simulink model "RollAxisAutopilotHarness"  (R2026a)
settings: Solver=FixedStepDiscrete  StartTime=0  StopTime=30  FixedStep=0.025
model workspace (MATLAB code in the model file):
  | cmdLim = Simulink.Parameter;
  | cmdLim.Value = 15;
  | cmdLim.Description = 'Limit for controlling the maximum surface command angle.';
  | cmdLim.Min = 0;
  | cmdLim.Max = 90;
  | cmdLim.DocUnits = 'deg';
  | 
  | dispGain = Simulink.Parameter;
  | dispGain.Value = 0.75;
  | dispGain.Description = 'Gain applied to the displacement error.';
  | dispGain.Min = 0;
  | dispGain.Max = [];
  | dispGain.DocUnits = 'deg/sec/deg';
  | 
  | dispLim = Simulink.Parameter;
  | dispLim.Value = 30;
  | dispLim.Description = 'Limit for controlling the maximum commanded angle.';
  | dispLim.Min = 0;
  | dispLim.Max = 180;
  | dispLim.DocUnits = 'deg';
  | 
  | intGain = Simulink.Parameter;
  | intGain.Value = 0.5;
  | intGain.Description = 'Gain applied to the integral error.';
  | intGain.Min = 0;
  | intGain.Max = [];
  | intGain.DocUnits = 'deg/sec/deg/sec';
  | 
  | intLim = Simulink.Parameter;
  | intLim.Value = 5;
  | intLim.Description = 'Limit for controlling the maximum commanded angle.';
  | intLim.Min = 0;
  | intLim.Max = 90;
  | intLim.DocUnits = 'deg';
  | 
  | rateGain = Simulink.Parameter;
  | rateGain.Value = 2;
  | rateGain.Description = 'Gain applied to the rate error.';
  | rateGain.Min = 0;
  | rateGain.Max = [];
  | rateGain.DocUnits = 'deg/deg/sec';
  | 
  | rateLim = Simulink.Parameter;
  | rateLim.Value = 6;
  | rateLim.Description = 'Limit for controlling the maximum commanded angle.';
  | rateLim.Min = 0;
  | rateLim.Max = 180;
  | rateLim.DocUnits = 'deg/sec';
  | 
  | hdgGain = Simulink.Parameter;
  | hdgGain.Value = 0.015;
libraries: SignalEditorBlockLib x1
settings Model: RequirementInfo={} %GIDa_fe9045fd_0412_4b6e_8206_617cc20e6fde  FPTRunName=Active  SldvGeneratedHarnessModel=TestUnitModel=rtwdemo_roll|  ModifiedByFormat=The MathWorks, Inc.  Creator=The MathWorks, Inc.  LastModifiedBy=The MathWorks, Inc.
settings DataIOCC: ExternalInput=xin  SaveFormat=StructureWithTime  OutputSaveName=harness_yout
settings OptimizationCC: UseDivisionForNetSlopeComputation=on  UseFloatMulNetSlope=on  InlineInvariantSignals=on  ExpressionFolding=off  StateBitsets=on  DataBitsets=on  EfficientFloat2IntCast=on  EfficientMapNaN2IntZero=off  MaxStackSize=inf
settings DebuggingCC: SignalRangeChecking=error  ReadBeforeWriteMsg=EnableAllAsError  WriteAfterWriteMsg=EnableAllAsError  WriteAfterReadMsg=EnableAllAsError  AlgebraicLoopMsg=error  ArtificialAlgebraicLoopMsg=error  SaveWithDisabledLinksMsg=error  SaveWithParameterizedLinksMsg=error  CheckExecutionContextPreStartOutputMsg=on  BlockPriorityViolationMsg=error  MaxConsecutiveZCsMsg=warning  SolverPrmCheckMsg=error  InheritedTsInSrcMsg=none  SingleTaskRateTransMsg=error  TasksWithSamePriorityMsg=error  SigSpecEnsureSampleTimeMsg=error  IntegerOverflowMsg=none  ParameterUnderflowMsg=error  ParameterPrecisionLossMsg=none  UnderSpecifiedDataTypeMsg=error  UnnecessaryDatatypeConvMsg=warning  VectorMatrixConversionMsg=error  SignalLabelMismatchMsg=error  UnconnectedInputMsg=error  UnconnectedOutputMsg=error  UnconnectedLineMsg=error  SFcnCompatibilityMsg=error  UniqueDataStoreMsg=error  BusObjectLabelMismatch=error  RootOutportRequireBusObject=error  AssertControl=DisableAll  ModelReferenceIOMismatchMessage=error  UnknownTsInhSupMsg=error  ModelReferenceDataLoggingMessage=error  ModelReferenceSymbolNameMessage=none  StrictBusMsg=ErrorOnBusTreatedAsVector  BusNameAdapt=ErrorWithoutRepair  NonBusSignalsTreatedAsBus=error  IntegerSaturationMsg=none
settings HardwareCC: TargetBitPerPointer=64.0  TargetBitPerSizeT=64.0  TargetBitPerPtrDiffT=64.0  TargetLongLongMode=on  TargetIntDivRoundTo=Zero  TargetEndianess=LittleEndian  TargetWordSize=64.0  TargetHWDeviceType=Custom Processor->MATLAB Host Computer  ProdEqTarget=off
settings RTWCC: SystemTargetFile=ert.tlc  GenerateReport=on  RTWVerbose=off  IncludeHyperlinkInReport=on  LaunchReport=on  Description=Embedded Coder
settings CodeAppCC: MATLABFcnDesc=on  MATLABSourceComments=on  EnableCustomComments=on  ReqsInCode=on
settings ERTTargetCC: DynamicArrayContainerType=coder::array  UtilityFuncGeneration=Shared location  MultiwordLength=2048.0  GenerateSampleERTMain=on  SupportContinuousTime=on
settings ConfigComp: CovSaveName=covdata_rollAP  CovMetricSettings=dcm  CovHTMLOptions=-sRT=1 -aTS=1 -bRG=1 -bTC=0 -hTR=0 -nFC=0 -scm=1 -bcm=1 -xEv=0  CovCumulativeVarName=covCumulativeData_rollAP  CovReportOnPause=off  DVMaxProcessTime=300.0  DVModelCoverageObjectives=MCDC  DVMaxTestCaseSteps=500.0  DVTestSuiteOptimization=Auto  DVAbsoluteTolerance=1.0e-5  DVDefectChecker=off  DVDetectActiveLogic=on  DVMaxViolationSteps=20.0  DVSaveHarnessModel=on  DVModelReferenceHarness=on  DVHarnessSource=Signal Editor  DVSaveReport=on  DVRebuildModelRepresentation=Always  DVActiveTab=0.0

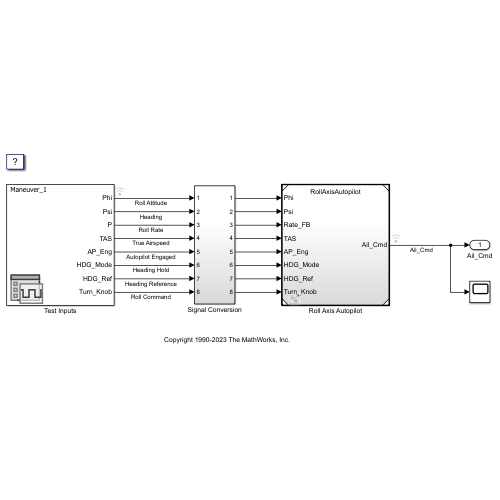
[thumbnail: Simulink's stored preview of the top-level diagram]
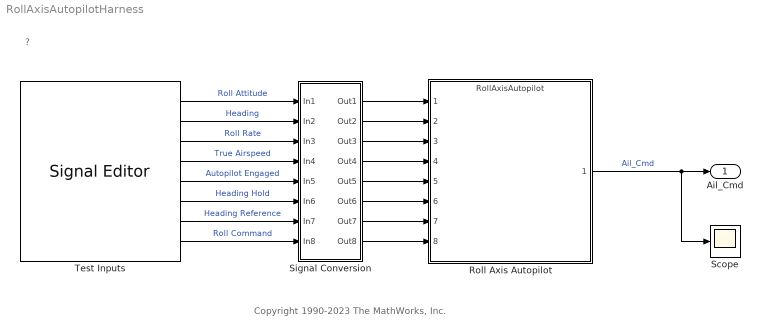
== system RollAxisAutopilotHarness ==
  note: Copyright 1990-2023 The MathWorks, Inc.
  note: ?
  Roll Axis Autopilot : ModelReference  ModelNameDialog=RollAxisAutopilot.slx  SimulationMode=Normal  ModelReferenceVersion=13.1
  Scope : Scope
      settings: DataLoggingSaveFormat=Array
  Signal Conversion : Subsystem
  Test Inputs : SignalEditorBlockLib/Signal Editor  FileName=roll_harness_TestInputs.mat  ActiveScenario=Maneuver_1  ActiveSignal=Turn_Knob  IsBus=off  OutputBusObjectStr=Bus: BusObject  SampleTime=0  ZeroCross=off  OutputAfterFinalValue=Extrapolation  Unit=inherit  PreserveSignalName=off  ApplySigPropsToAllScenarios=on  ApplySigPropsToAllSignals=off  SignalPropertySource=Dialog parameters
  Ail_Cmd : Outport  RequirementInfo={} %GIDa_7d37a828_8c9c_441a_973a_3dcc496ec4f2  OutMin=-15  OutMax=15  OutDataTypeStr=single  PortDimensions=1  SampleTime=1/40  VectorParamsAs1DForOutWhenUnconnected=off
  wires:
  Test Inputs/1 -> Signal Conversion/1(In1)  "Roll Attitude"
  Signal Conversion/1(Out1) -> Roll Axis Autopilot/1
  Test Inputs/2 -> Signal Conversion/2(In2)  "Heading"
  Signal Conversion/2(Out2) -> Roll Axis Autopilot/2
  Test Inputs/3 -> Signal Conversion/3(In3)  "Roll Rate"
  Signal Conversion/3(Out3) -> Roll Axis Autopilot/3
  Test Inputs/4 -> Signal Conversion/4(In4)  "True Airspeed"
  Signal Conversion/4(Out4) -> Roll Axis Autopilot/4
  Test Inputs/5 -> Signal Conversion/5(In5)  "Autopilot Engaged"
  Signal Conversion/5(Out5) -> Roll Axis Autopilot/5
  Test Inputs/6 -> Signal Conversion/6(In6)  "Heading Hold"
  Signal Conversion/6(Out6) -> Roll Axis Autopilot/6
  Test Inputs/7 -> Signal Conversion/7(In7)  "Heading Reference"
  Signal Conversion/7(Out7) -> Roll Axis Autopilot/7
  Test Inputs/8 -> Signal Conversion/8(In8)  "Roll Command"
  Signal Conversion/8(Out8) -> Roll Axis Autopilot/8
  Roll Axis Autopilot/1 -> Scope/1, Ail_Cmd/1  "Ail_Cmd"

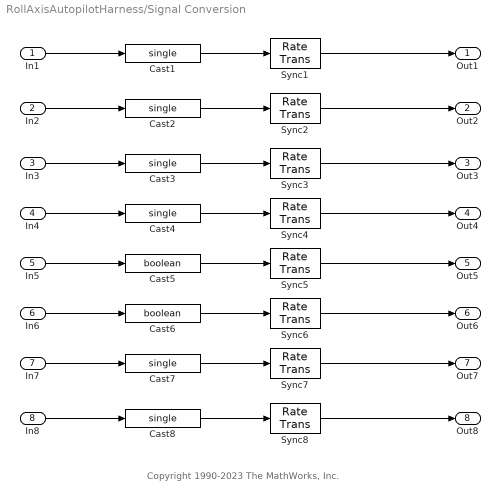
== system RollAxisAutopilotHarness/Signal Conversion ==
  note: Copyright 1990-2023 The MathWorks, Inc.
  In1 : Inport
  In2 : Inport  Port=2
  In3 : Inport  Port=3
  In4 : Inport  Port=4
  In5 : Inport  Port=5
  In6 : Inport  Port=6
  In7 : Inport  Port=7
  In8 : Inport  Port=8
  Cast{1..4,7..8} (6 alike) : DataTypeConversion  OutDataTypeStr=single
  Cast5 : DataTypeConversion  OutDataTypeStr=boolean
  Cast6 : DataTypeConversion  OutDataTypeStr=boolean
  Sync{1..8} (8 alike) : RateTransition  OutPortSampleTime=[0.025,0]
  Out1 : Outport  VectorParamsAs1DForOutWhenUnconnected=off
  Out2 : Outport  Port=2  VectorParamsAs1DForOutWhenUnconnected=off
  Out3 : Outport  Port=3  VectorParamsAs1DForOutWhenUnconnected=off
  Out4 : Outport  Port=4  VectorParamsAs1DForOutWhenUnconnected=off
  Out5 : Outport  Port=5  VectorParamsAs1DForOutWhenUnconnected=off
  Out6 : Outport  Port=6  VectorParamsAs1DForOutWhenUnconnected=off
  Out7 : Outport  Port=7  VectorParamsAs1DForOutWhenUnconnected=off
  Out8 : Outport  Port=8  VectorParamsAs1DForOutWhenUnconnected=off
  wires:
  In1/1 -> Cast1/1
  Cast1/1 -> Sync1/1
  Sync1/1 -> Out1/1
  In2/1 -> Cast2/1
  Cast2/1 -> Sync2/1
  Sync2/1 -> Out2/1
  In3/1 -> Cast3/1
  Cast3/1 -> Sync3/1
  Sync3/1 -> Out3/1
  In4/1 -> Cast4/1
  Cast4/1 -> Sync4/1
  Sync4/1 -> Out4/1
  In5/1 -> Cast5/1
  Cast5/1 -> Sync5/1
  Sync5/1 -> Out5/1
  In6/1 -> Cast6/1
  Cast6/1 -> Sync6/1
  Sync6/1 -> Out6/1
  In7/1 -> Cast7/1
  Cast7/1 -> Sync7/1
  Sync7/1 -> Out7/1
  In8/1 -> Cast8/1
  Cast8/1 -> Sync8/1
  Sync8/1 -> Out8/1
